simulink model "estado"  (R2013a)
settings: Solver=ode45  StartTime=0.0  StopTime=10.0  RelTol=1e-3
settings Model: Creator=juliocesar  LastModifiedBy=Alejandro
settings DataIOCC: SignalLoggingSaveFormat=ModelDataLogs
settings DebuggingCC: UnderspecifiedInitializationDetection=Simplified  MultiTaskDSMMsg=warning  MultiTaskCondExecSysMsg=none  StateNameClashWarn=none  StrictBusMsg=None
settings RTWCC: IncludeERTFirstTime=on
settings GRTTargetCC: CodeReplacementLibrary=None  CPPClassGenCompliant=on

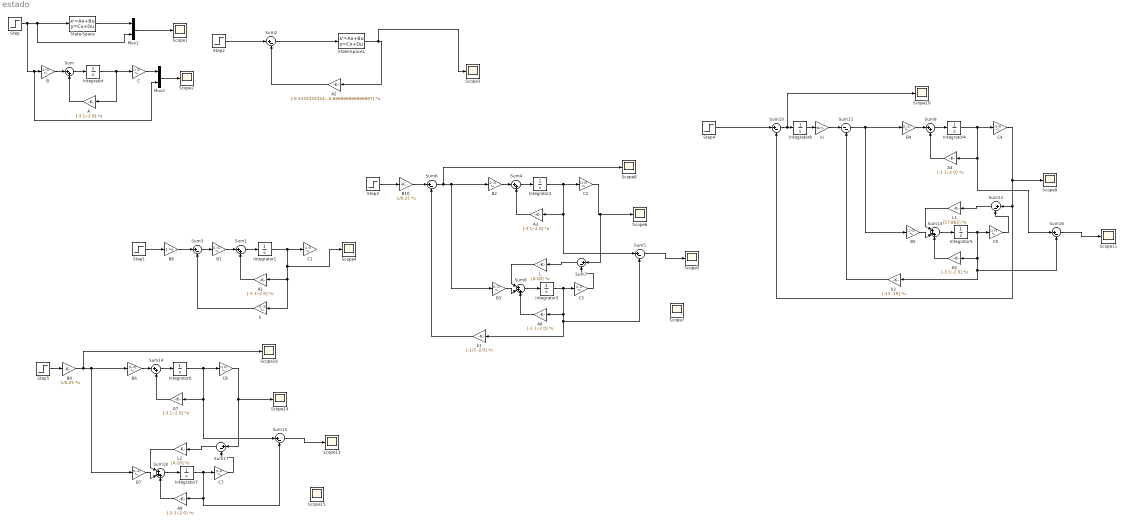
== system estado ==
  A{,1,3..8} (8 alike) : Gain  Gain=[-3 1;-2 0]  Multiplication=Matrix(K*u)
  A2 : Gain  Gain=[-0.333333333333333 -0.666666666666667]  Multiplication=Matrix(K*u)
  B{,1..7} (8 alike) : Gain  Gain=[1;-2]  Multiplication=Matrix(K*u)
  B10 : Gain  Gain=-1/0.25  Multiplication=Matrix(K*u)
  B8 : Gain  Multiplication=Matrix(K*u)
  B9 : Gain  Gain=-1/0.25  Multiplication=Matrix(K*u)
  C{,1..7} (8 alike) : Gain  Gain=[1 0]  Multiplication=Matrix(K*u)
  Integrator{,1..3,5,7..8} (7 alike) : Integrator
  Integrator4 : Integrator  InitialCondition=10
  Integrator6 : Integrator  InitialCondition=10
  L : Gain  Gain=[4;10]  Multiplication=Matrix(K*u)
  L1 : Gain  Gain=[57;862]  Multiplication=Matrix(K*u)
  L2 : Gain  Gain=[4;10]  Multiplication=Matrix(K*u)
  Mux1 : Mux  Inputs=2
  Mux2 : Mux  Inputs=2
  Scope{1..11,13..16} (15 alike) : Scope
      Scope10 settings: SaveName=ScopeData9  SampleInput=on  SampleTime=0.01
      Scope11 settings: SaveName=ScopeData10  SampleTime=0.01
      Scope13 settings: SaveName=ScopeData12  SampleInput=on  SampleTime=0.01
      Scope14 settings: SaveName=ScopeData13  SampleInput=on  SampleTime=0.01
      Scope15 settings: SaveName=ScopeData14  SampleInput=on  SampleTime=0.01
      Scope16 settings: SaveName=ScopeData15  SampleInput=on  SampleTime=0.01
      Scope3 settings: SaveName=ScopeData2
      Scope4 settings: SaveName=ScopeData3  SampleInput=on  SampleTime=0.01
      Scope5 settings: SaveName=ScopeData4  SampleInput=on  SampleTime=0.01
      Scope6 settings: SaveName=ScopeData5  SampleInput=on  SampleTime=0.01
      Scope7 settings: SaveName=ScopeData6  SampleInput=on  SampleTime=0.01
      Scope8 settings: SaveName=ScopeData7  SampleInput=on  SampleTime=0.01
      Scope9 settings: SaveName=ScopeData8  SampleInput=on  SampleTime=0.01
  State-Space : StateSpace  A=[-3 1; -2 0]  B=[1; -2]  C=[1 0]  D=0
  State-Space1 : StateSpace  A=[-3 1; -2 0]  B=[1; -2]  C=[1 0;0 0]  D=[0;0]
  Step : Step  SampleTime=0
  Step1 : Step  SampleTime=0
  Step2 : Step  SampleTime=0
  Step3 : Step  Time=0  SampleTime=0
  Step4 : Step  Time=5  SampleTime=0
  Step5 : Step  Time=0  SampleTime=0
  Sum{,1,4,9,14} (5 alike) : Sum  Inputs=|++
  Sum{2..3,5..7,10,12,15..17} (10 alike) : Sum  Inputs=|+-
  Sum11 : Sum  Inputs=|--
  Sum13 : Sum  Inputs=|+++
  Sum18 : Sum  Inputs=|+++
  Sum8 : Sum  Inputs=|+++
  k : Gain  Gain=[1 -3]  Multiplication=Matrix(K*u)
  k1 : Gain  Gain=[-1/3 -2/3]  Multiplication=Matrix(K*u)
  k2 : Gain  Gain=[-23 -19]  Multiplication=Matrix(K*u)
  ki : Gain  Gain=96  Multiplication=Matrix(K*u)
  wires:
  Step/1 -> Mux2/2, B/1, Mux1/2, State-Space/1
  Mux1/1 -> Scope1/1
  State-Space/1 -> Mux1/1
  Integrator/1 -> A/1, C/1
  Sum/1 -> Integrator/1
  A/1 -> Sum/2
  B/1 -> Sum/1
  Mux2/1 -> Scope2/1
  C/1 -> Mux2/1
  State-Space1/1 -> Scope3/1, A2/1
  Sum2/1 -> State-Space1/1
  A2/1 -> Sum2/2
  Sum1/1 -> Integrator1/1
  A1/1 -> Sum1/2
  B1/1 -> Sum1/1
  Sum3/1 -> B1/1
  k/1 -> Sum3/2
  Integrator1/1 -> C1/1, Scope4/1, k/1, A1/1
  Step1/1 -> B8/1
  Step2/1 -> Sum2/1
  Sum8/1 -> Integrator3/1
  C3/1 -> Sum7/2
  A6/1 -> Sum8/3
  B3/1 -> Sum8/2
  Sum7/1 -> L/1
  L/1 -> Sum8/1
  Sum4/1 -> Integrator2/1
  A3/1 -> Sum4/2
  B2/1 -> Sum4/1
  Integrator3/1 -> Sum5/2, k1/1, A6/1, C3/1
  Sum5/1 -> Scope5/1
  Integrator2/1 -> Sum5/1, A3/1, C2/1
  C2/1 -> Scope6/1, Sum7/1
  k1/1 -> Sum6/2
  Step3/1 -> B10/1
  Sum6/1 -> B2/1, B3/1, Scope8/1
  Sum13/1 -> Integrator5/1
  C5/1 -> Sum12/2
  A5/1 -> Sum13/3
  B5/1 -> Sum13/2
  Sum12/1 -> L1/1
  L1/1 -> Sum13/1
  Sum9/1 -> Integrator4/1
  A4/1 -> Sum9/2
  B4/1 -> Sum9/1
  Integrator5/1 -> Sum16/2, k2/1, A5/1, C5/1
  Integrator4/1 -> Sum16/1, A4/1, C4/1
  C4/1 -> Scope9/1, Sum10/2, Sum12/1
  k2/1 -> Sum11/2
  Sum11/1 -> B4/1, B5/1
  Sum18/1 -> Integrator7/1
  C7/1 -> Sum17/2
  A8/1 -> Sum18/3
  B7/1 -> Sum18/2
  Sum17/1 -> L2/1
  L2/1 -> Sum18/1
  Sum14/1 -> Integrator6/1
  A7/1 -> Sum14/2
  B6/1 -> Sum14/1
  Integrator7/1 -> Sum15/2, A8/1, C7/1
  Sum15/1 -> Scope13/1
  Integrator6/1 -> Sum15/1, A7/1, C6/1
  C6/1 -> Scope14/1, Sum17/1
  Step5/1 -> B9/1
  B8/1 -> Sum3/1
  B9/1 -> B6/1, B7/1, Scope16/1
  B10/1 -> Sum6/1
  Integrator8/1 -> ki/1
  ki/1 -> Sum11/1
  Step4/1 -> Sum10/1
  Sum10/1 -> Scope10/1, Integrator8/1
  Sum16/1 -> Scope11/1
